simulink model "task1"  (R2024a)
settings: Solver=VariableStepAuto  StartTime=0.0  StopTime=10.0  MaxStep=0.001  RelTol=1e-3
undefined symbols (not defined in the file): Abar, Bbar, C, D, e0_bar, Gamma_g, Gbar, K, wg0, Yg
settings Model: Creator=sizgr  LastModifiedBy=sizgr

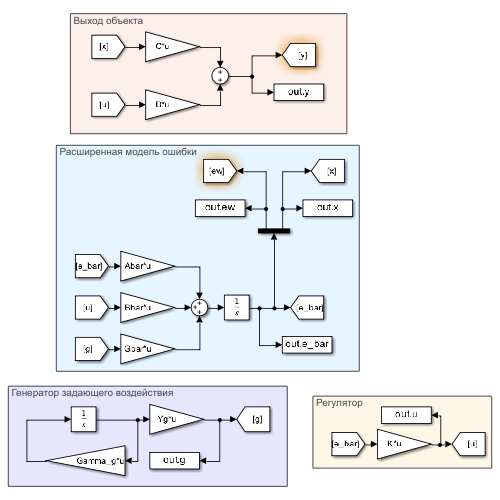
[thumbnail: Simulink's stored preview of the top-level diagram]
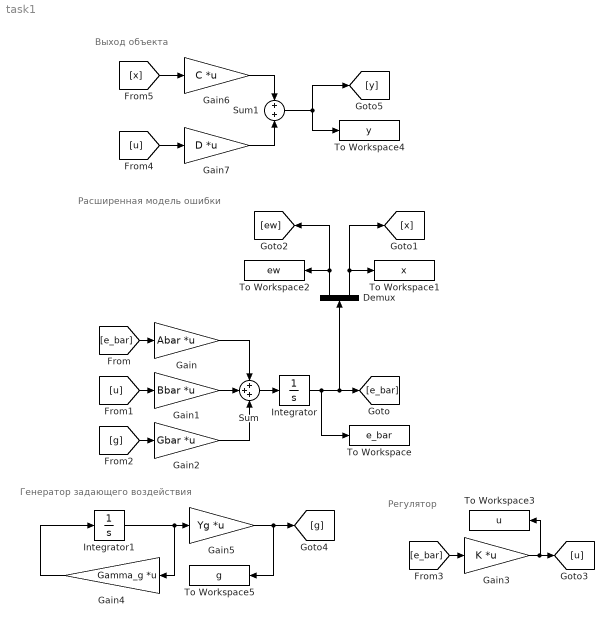
== system task1 ==
  note: Выход объекта
  note: Генератор задающего воздействия
  note: Регулятор
  note: Расширенная модель ошибки
  Demux : Demux  Outputs=2
  Gain : Gain  Gain=Abar  Multiplication=Matrix(K*u)
  Gain1 : Gain  Gain=Bbar  Multiplication=Matrix(K*u)
  Gain2 : Gain  Gain=Gbar  Multiplication=Matrix(K*u)
  Gain3 : Gain  Gain=K  Multiplication=Matrix(K*u)
  Gain4 : Gain  Gain=Gamma_g  Multiplication=Matrix(K*u)
  Gain5 : Gain  Gain=Yg  Multiplication=Matrix(K*u)
  Gain6 : Gain  Gain=C  Multiplication=Matrix(K*u)
  Gain7 : Gain  Gain=D  Multiplication=Matrix(K*u)
  Integrator : Integrator  InitialCondition=e0_bar
  Integrator1 : Integrator  InitialCondition=wg0
  Sum : Sum  Inputs=+++
  Sum1 : Sum  Inputs=+|+
  To Workspace : ToWorkspace  VariableName=e_bar  SaveFormat=Timeseries  SampleTime=-1
  To Workspace1 : ToWorkspace  VariableName=x  SaveFormat=Timeseries  SampleTime=-1
  To Workspace2 : ToWorkspace  VariableName=ew  SaveFormat=Timeseries  SampleTime=-1
  To Workspace3 : ToWorkspace  VariableName=u  SaveFormat=Timeseries  SampleTime=-1
  To Workspace4 : ToWorkspace  VariableName=y  SaveFormat=Timeseries  SampleTime=-1
  To Workspace5 : ToWorkspace  VariableName=g  SaveFormat=Timeseries  SampleTime=-1
  wires:
  Sum/1 -> Integrator/1
  Integrator/1 -> Demux/1, [e_bar], To Workspace/1
  [e_bar] -> Gain/1
  [u] -> Gain1/1
  [g] -> Gain2/1
  Gain1/1 -> Sum/2
  Gain/1 -> Sum/1
  Gain2/1 -> Sum/3
  Demux/2 -> To Workspace1/1, [x]
  Demux/1 -> To Workspace2/1, [ew]
  [e_bar] -> Gain3/1
  Gain3/1 -> To Workspace3/1, [u]
  Integrator1/1 -> Gain5/1, Gain4/1
  Gain4/1 -> Integrator1/1
  Gain5/1 -> [g], To Workspace5/1
  Gain6/1 -> Sum1/1
  Gain7/1 -> Sum1/2
  [u] -> Gain7/1
  [x] -> Gain6/1
  Sum1/1 -> To Workspace4/1, [y]
